simulink model "three_phase_ac_voltage_controller"  (R2023b)
settings: Solver=ode45  StartTime=0.0  StopTime=0.5  RelTol=1e-5  EnableMultiTasking=on
libraries: spsVoltageMeasurementLib x6, spsThyristorLib x6, spsACVoltageSourceLib x3, spsCurrentMeasurementLib x3, spsGroundLib x2, spsThreePhaseSeriesRLCBranchLib x1, spspowerguiLib x1
Description:
  | Created By:
  | Uvesh Sipai
  | For any further help regarding this contact me on : uvesh.sipai [at] gmail.com
settings Model: Creator=Uvesh Sipai  LastModifiedBy=dhana
settings SolverCC: AlgebraicLoopSolver=TrustRegion
settings DataIOCC: LimitDataPoints=on  SaveFormat=Array  ReturnWorkspaceOutputs=off
settings OptimizationCC: LifeSpan=inf
settings DebuggingCC: SolverPrmCheckMsg=warning  UnconnectedInputMsg=warning  UnconnectedOutputMsg=warning  UnconnectedLineMsg=warning  SFUnexpectedBacktrackingDiag=warning  SFNoUnconditionalDefaultTransitionDiag=warning  SFExecutionAtInitializationDiag=none  ArithmeticOperatorsInVariantConditions=warning
settings HardwareCC: ProdBitPerPointer=32  ProdBitPerSizeT=32  ProdBitPerPtrDiffT=32  ProdLargestAtomicFloat=None  ProdIntDivRoundTo=Undefined  ProdEndianess=Unspecified  ProdWordSize=32  ProdHWDeviceType=32-bit Generic
settings ModelReferenceCC: PropagateSignalLabelsOutOfModel=off
settings SFSimCC: SimUseLocalCustomCode=off  CustomCodeUndefinedFunction=UseInterfaceOnly
settings RTWCC: RTWUseLocalCustomCode=off
settings CodeAppCC: StateflowObjectComments=on
settings GRTTargetCC: TargetLangStandard=C89/C90 (ANSI)
settings ConfigComp: CovMetricSettings=dw  CovSaveCumulativeToWorkspaceVar=on  CovSaveSingleToWorkspaceVar=on  CovExternalEMLEnable=off  CovSFcnEnable=off
settings SimscapeCC: SimscapeNormalizeSystem=off

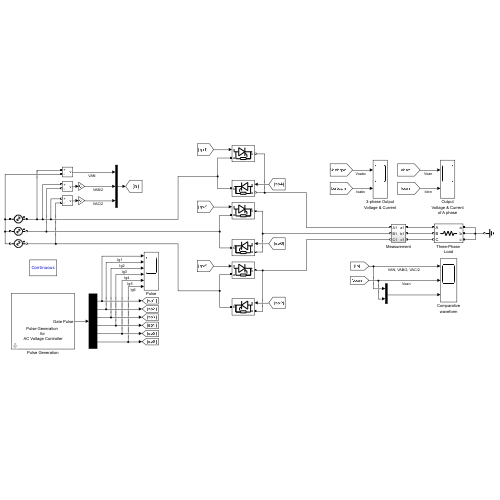
[thumbnail: Simulink's stored preview of the top-level diagram]
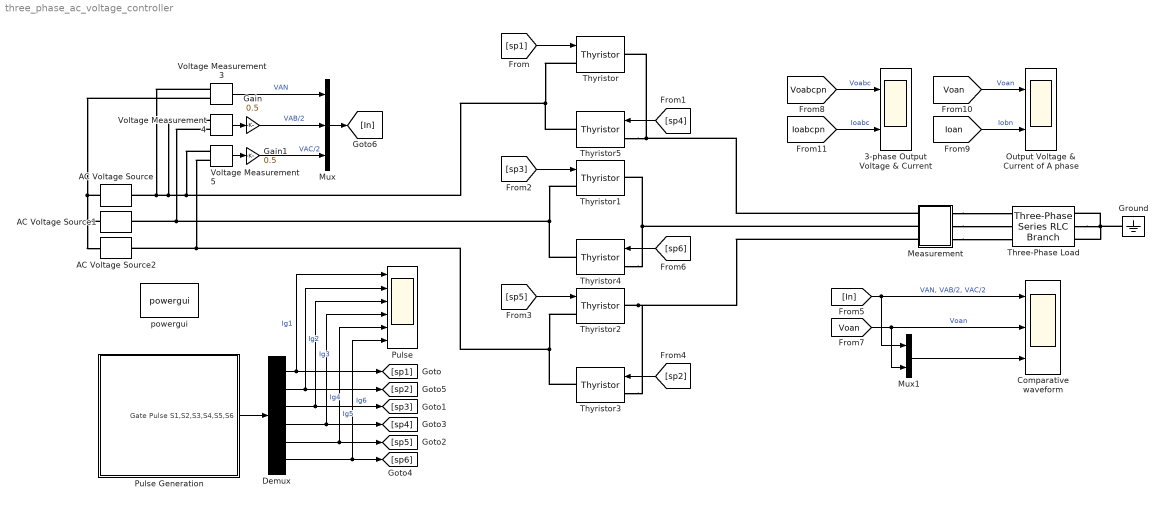
== system three_phase_ac_voltage_controller ==
  3-phase Output Voltage & Current : Scope  NumInputPorts=2
  AC Voltage Source : spsACVoltageSourceLib/AC Voltage Source  Amplitude=339.4113  Phase=0  Frequency=50  SampleTime=0  Measurements=Voltage  BusType=swing  Pref=10e3  Qref=0  Qmin=-inf  Qmax=+inf
  AC Voltage Source1 : spsACVoltageSourceLib/AC Voltage Source  Amplitude=339.4113  Phase=-120  Frequency=50  SampleTime=0  Measurements=Voltage  BusType=swing  Pref=10e3  Qref=0  Qmin=-inf  Qmax=+inf
  AC Voltage Source2 : spsACVoltageSourceLib/AC Voltage Source  Amplitude=339.4113  Phase=120  Frequency=50  SampleTime=0  Measurements=Voltage  BusType=swing  Pref=10e3  Qref=0  Qmin=-inf  Qmax=+inf
  Comparative waveform : Scope  NumInputPorts=3
  Demux : Demux  Outputs=6
  Gain : Gain  Gain=0.5
  Gain1 : Gain  Gain=0.5
  Ground : spsGroundLib/Ground  LConnTagsString=a
  Measurement : Subsystem
  Mux : Mux  Inputs=3
  Mux1 : Mux  Inputs=2
  Output Voltage & Current of A phase : Scope  NumInputPorts=2
  Pulse : Scope  NumInputPorts=6
  Pulse Generation : Subsystem  mask{con=Integral Cycle Control with Phase Angle control, freq=50, alpha=54.0, n=3, m=2}
      mask prompts: con "Type of Control"; freq "Operating Frequency"; alpha "Firing Angle (Alpha)"; n "Number of ON cycle (n)"; m "Number of OFF cycle (m)"
      mask init:
      | if con==1
      |     tpf=1/freq;
      |     delay=alpha;
      |     if alpha<120
      |         pw=((180-alpha)/360)*100;
      |     else
      |         pw=((180-alpha+30)/360)*100;
      |     end
      |     tpfin=tpf;
      |     pwin=99.9999999999;
      |     delayin=0;
      | elseif con==2
      |     tpf=1/freq;
      |     delay=0;
      |     pw=50;
      |     tpfin=(m+n)*tpf;
      |     pwin=(n/(m+n))*100;
      |     delayin=0;
      | else
      |     tpf=1/freq;
      |     delay=alpha;
      |     if alpha<120
      |         pw=((180-alpha)/360)*100;
      |     else
      |         pw=((180-alpha+30)/360)*100;
      |     end
      |     tpfin=(m+n)*tpf;
      |     pwin=(n/(m+n))*100;
      |     delayin=0;
      | end
      | 
      |     %alpha with alpha=0 at wt=0
      mask Help:
      | This Block is use for pulse generation for Three Phase AC voltage controller.
      | By varying the operating frequency one can vary the operating frequency.
      | By varying the Firing angle by knob, the firing angle is vary.
      | By changing the value of number of on cycle(n) and number of off cycle(m), output is vary in intigral cycle control.
      | Also there is two possible mode of Operation (1)Phase Angle Control (2)Integral cycle control (3)Intigral Cycle Control with Phase angle control
      | When Phase Angle control is selected then the effect of number of on cycle and no of off cycle is not there. And same when Integral cycle control
      | is selected then effect of firing angle is not there. When the Integral Cycle control with Phase angle control is selected at that time effect of
      | both number of on/off cycle and firing angle is there.
      | 
      | Created By:
      | Uvesh Sipai
      | For any further help regarding this contact me on : uvesh.sipai [at] gmail.com
      mask TypeOptions con: Phase Angle Control | Intigral Cycle Control | Integral Cycle Control with Phase Angle control
      mask DialogControl DescGroupVar Prompt: Pulse Generation for Three Phase AC voltage controller
      mask DialogControl DescTextVar Prompt: This Block is use for pulse generation for Three Phase AC voltage controller.  Also there are three possible mode of operation.
      mask DialogControl DescTextVar_copy Prompt: Made by : Uvesh Sipai
      mask DialogControl Control4 Prompt: For more help contact me on : uvesh.sipai [at] gmail.com
      mask DialogControl linkoffb Prompt: https://www.facebook.com/uvesh.sipai
      mask DialogControl Container6 Prompt: Parameter for Phase Angle control
      mask DialogControl intigral Prompt: Parameter for Integral Cycle control
      mask Display:
      | disp('\n \n \n \n \nPulse Generation \n for \n AC Voltage Controller')
      | %disp('\n \n \n \n \n by Uvesh Sipai')
      | port_label('output', 1, 'Gate Pulse')
  Three-Phase Load : spsThreePhaseSeriesRLCBranchLib/Three-Phase Series RLC Branch  LConnTagsString=A|B|C  RConnTagsString=A|B|C  BranchType=R  Resistance=1  Inductance=1e-3  Capacitance=1e-6  Measurements=None
  Thyristor{,1..5} (6 alike) : spsThyristorLib/Thyristor  Ron=0.001  Lon=0  Vf=0.8  IC=0  Rs=500  Cs=250e-9  Measurements=off
  Voltage Measurement3 : spsVoltageMeasurementLib/Voltage Measurement  PhasorSimulation=off  OutputType=Complex  PSBequivalent=0
  Voltage Measurement4 : spsVoltageMeasurementLib/Voltage Measurement  PhasorSimulation=off  OutputType=Complex  PSBequivalent=0
  Voltage Measurement5 : spsVoltageMeasurementLib/Voltage Measurement  PhasorSimulation=off  OutputType=Complex  PSBequivalent=0
  powergui : spspowerguiLib/powergui  Priority=1  SimulationMode=Continuous  SampleTime=50e-6  frequency=60  Iterations=50  frequencyindice=0  Pbase=100e6  ErrMax=1e-4  UnitsV=kV  UnitsW=MW  buscounter=0  FunctionMessages=off  echomessages=off  EnableUseOfTLC=off  CurrentSourceSwitches=off  DisableSnubberDevices=off  DisableRonSwitches=off  DisableVfSwitches=off  DisplayEquations=off  AutomaticDiscreteSolvers=off  SolverType=Tustin  Interpol=off  ExternalGateDelay=off  methode=off  Ts=0  x0status=blocks  SPID=off  SwTol=0  HookPort=off  NonlinearTolerance=1e-4  nMaxIteration=100  ContinueOnMaxIteration=off  RestoreLinks=warning  ResistiveCurrentMeasurement=off  Frange=[0:2:500]  Ylog=off  Xlog=on  ShowGrid=off  save=off  variable=ZData  structure=0  ZoomFFT=off  StartTime=0.0  cycles=1  DisplayStyle=1  fundamental=60  FreqAxis=off  MaxFrequency=1000  frequencyindicesteady=1  RmsSteady=1  display=off
  wires:
  [sp1] -> Thyristor/1
  [sp4] -> Thyristor5/1
  [sp3] -> Thyristor1/1
  [sp6] -> Thyristor4/1
  [sp5] -> Thyristor2/1
  [sp2] -> Thyristor3/1
  Voltage Measurement4/1 -> Gain/1
  Voltage Measurement5/1 -> Gain1/1
  Voltage Measurement3/1 -> Mux/1  "VAN"
  Gain/1 -> Mux/2  "VAB/2"
  Gain1/1 -> Mux/3  "VAC/2"
  Mux/1 -> [In]
  [In] -> Comparative waveform/1, Mux1/1  "VAN, VAB/2, VAC/2"
  [Voan] -> Mux1/2, Comparative waveform/2  "Voan"
  [Voabcpn] -> 3-phase Output Voltage & Current/1  "Voabc"
  [Ioabcpn] -> 3-phase Output Voltage & Current/2  "Ioabc"
  Mux1/1 -> Comparative waveform/3
  Demux/1 -> Pulse/1, [sp1]  "Ig1"
  Demux/2 -> Pulse/2, [sp2]  "Ig2"
  Demux/3 -> Pulse/3, [sp3]  "Ig3"
  Demux/4 -> Pulse/4, [sp4]  "Ig4"
  Demux/5 -> Pulse/5, [sp5]  "Ig5"
  Demux/6 -> [sp6], Pulse/6  "Ig6"
  Pulse Generation/1(Gate Pulse S1,S2,S3,S4,S5,S6) -> Demux/1
  [Voan] -> Output Voltage & Current of A phase/1  "Voan"
  [Ioan] -> Output Voltage & Current of A phase/2  "Iobn"
  connections:
  Thyristor/LConn1 -- Voltage Measurement5/LConn1 -- Voltage Measurement4/LConn1 -- Voltage Measurement3/LConn1 -- AC Voltage Source/RConn1 -- Thyristor5/RConn1
  Thyristor1/LConn1 -- Thyristor4/RConn1 -- Voltage Measurement4/LConn2 -- AC Voltage Source1/RConn1
  Three-Phase Load/RConn2 -- Ground/LConn1 -- Three-Phase Load/RConn3 -- Three-Phase Load/RConn1
  Thyristor2/LConn1 -- AC Voltage Source2/RConn1 -- Voltage Measurement5/LConn2 -- Thyristor3/RConn1
  AC Voltage Source/LConn1 -- AC Voltage Source2/LConn1 -- AC Voltage Source1/LConn1 -- Voltage Measurement3/LConn2
  Thyristor5/LConn1 -- Measurement/LConn1 -- Thyristor/RConn1
  Thyristor4/LConn1 -- Measurement/LConn2 -- Thyristor1/RConn1
  Thyristor2/RConn1 -- Measurement/LConn3 -- Thyristor3/LConn1
  Measurement/RConn1 -- Three-Phase Load/LConn1
  Measurement/RConn2 -- Three-Phase Load/LConn2
  Measurement/RConn3 -- Three-Phase Load/LConn3

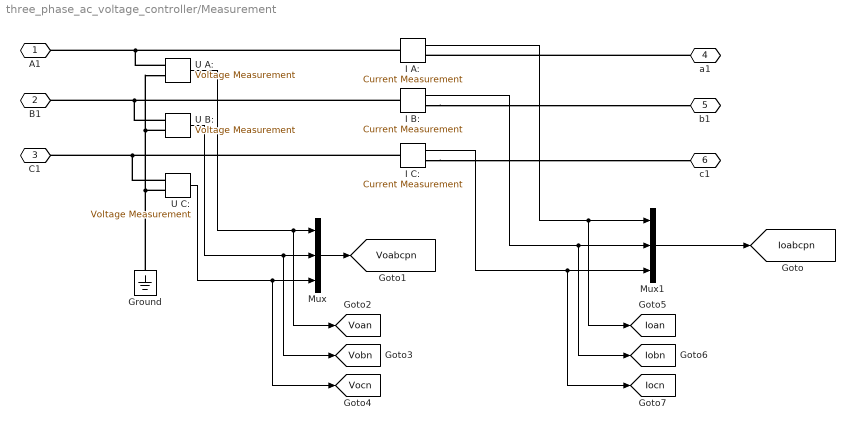
== system three_phase_ac_voltage_controller/Measurement ==
  Ground : spsGroundLib/Ground  LConnTagsString=a
  I A: : spsCurrentMeasurementLib/Current Measurement  PhasorSimulation=off  OutputType=Complex  PSBequivalent=0
  I B: : spsCurrentMeasurementLib/Current Measurement  PhasorSimulation=off  OutputType=Complex  PSBequivalent=0
  I C: : spsCurrentMeasurementLib/Current Measurement  PhasorSimulation=off  OutputType=Complex  PSBequivalent=0
  Mux : Mux  Inputs=3
  Mux1 : Mux  Inputs=3
  U A: : spsVoltageMeasurementLib/Voltage Measurement  PhasorSimulation=off  OutputType=Complex  PSBequivalent=0
  U B: : spsVoltageMeasurementLib/Voltage Measurement  PhasorSimulation=off  OutputType=Complex  PSBequivalent=0
  U C: : spsVoltageMeasurementLib/Voltage Measurement  PhasorSimulation=off  OutputType=Complex  PSBequivalent=0
  A1 : PMIOPort  Side=Left
  B1 : PMIOPort  Port=2  Side=Left
  C1 : PMIOPort  Port=3  Side=Left
  a1 : PMIOPort  Port=4  Side=Right
  b1 : PMIOPort  Port=5  Side=Right
  c1 : PMIOPort  Port=6  Side=Right
  tag scope: Ioabcpn=global, Ioan=global, Iobn=global, Iocn=global, Voabcpn=global, Voan=global, Vobn=global, Vocn=global
  wires:
  U A:/1 -> [Voan], Mux/1
  U B:/1 -> [Vobn], Mux/2
  Mux1/1 -> [Ioabcpn]
  Mux/1 -> [Voabcpn]
  U C:/1 -> [Vocn], Mux/3
  I A:/1 -> [Ioan], Mux1/1
  I B:/1 -> [Iobn], Mux1/2
  I C:/1 -> [Iocn], Mux1/3
  connections:
  a1/RConn1 -- I A:/RConn1
  I C:/LConn1 -- U C:/LConn1 -- C1/RConn1
  U C:/LConn2 -- U B:/LConn2 -- U A:/LConn2 -- Ground/LConn1
  I C:/RConn1 -- c1/RConn1
  I B:/LConn1 -- U B:/LConn1 -- B1/RConn1
  I B:/RConn1 -- b1/RConn1
  I A:/LConn1 -- U A:/LConn1 -- A1/RConn1

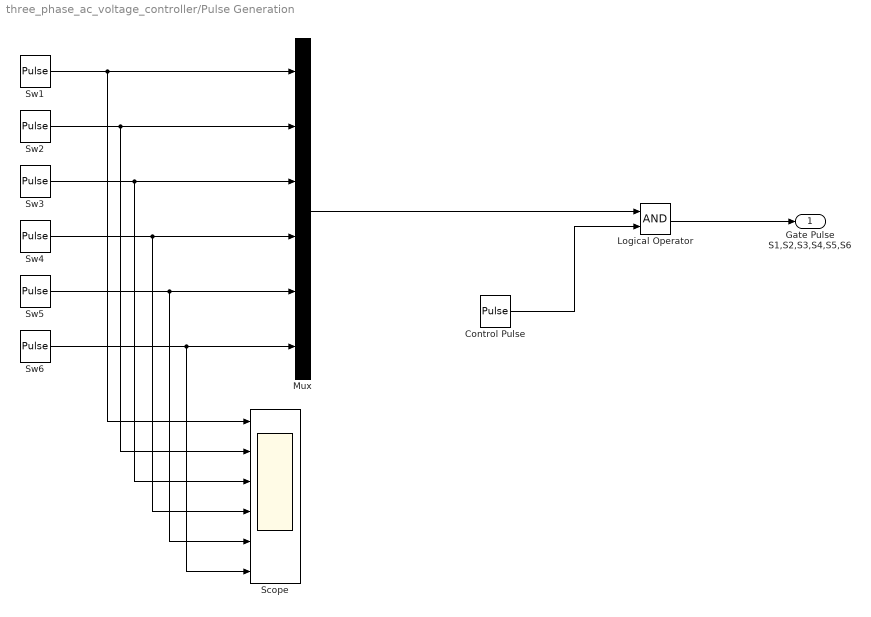
== system three_phase_ac_voltage_controller/Pulse Generation ==
  Control Pulse : DiscretePulseGenerator  PulseType=Time based  Period=tpfin  PulseWidth=pwin  PhaseDelay=delayin
  Logical Operator : Logic  AllPortsSameDT=off  OutDataTypeStr=boolean
  Mux : Mux  Inputs=6
  Scope : Scope  NumInputPorts=6
  Sw1 : DiscretePulseGenerator  PulseType=Time based  Period=tpf  PulseWidth=pw  PhaseDelay=(delay)*(tpf/360)
  Sw2 : DiscretePulseGenerator  PulseType=Time based  Period=tpf  PulseWidth=pw  PhaseDelay=(delay+60)*(tpf/360)
  Sw3 : DiscretePulseGenerator  PulseType=Time based  Period=tpf  PulseWidth=pw  PhaseDelay=(delay+120)*(tpf/360)
  Sw4 : DiscretePulseGenerator  PulseType=Time based  Period=tpf  PulseWidth=pw  PhaseDelay=(delay+180)*(tpf/360)
  Sw5 : DiscretePulseGenerator  PulseType=Time based  Period=tpf  PulseWidth=pw  PhaseDelay=(delay-120)*(tpf/360)
  Sw6 : DiscretePulseGenerator  PulseType=Time based  Period=tpf  PulseWidth=pw  PhaseDelay=(delay-60)*(tpf/360)
  Gate Pulse S1,S2,S3,S4,S5,S6 : Outport
  wires:
  Sw1/1 -> Scope/1, Mux/1
  Sw2/1 -> Scope/2, Mux/2
  Sw3/1 -> Scope/3, Mux/3
  Sw4/1 -> Scope/4, Mux/4
  Sw5/1 -> Scope/5, Mux/5
  Sw6/1 -> Scope/6, Mux/6
  Mux/1 -> Logical Operator/1
  Control Pulse/1 -> Logical Operator/2
  Logical Operator/1 -> Gate Pulse S1,S2,S3,S4,S5,S6/1
